simulink model "projectinitial-1"  (R2016a)
settings: Solver=VariableStepAuto  StartTime=0.0  StopTime=0.2  RelTol=1e-3
undefined symbols (not defined in the file): D1, Delta
libraries: powerlib x27, simulink_extras x2, dspsigops x2, powerlib_meascontrol x2
settings Model: Creator=Ejapistic Aamir  LastModifiedBy=Ejapistic Aamir

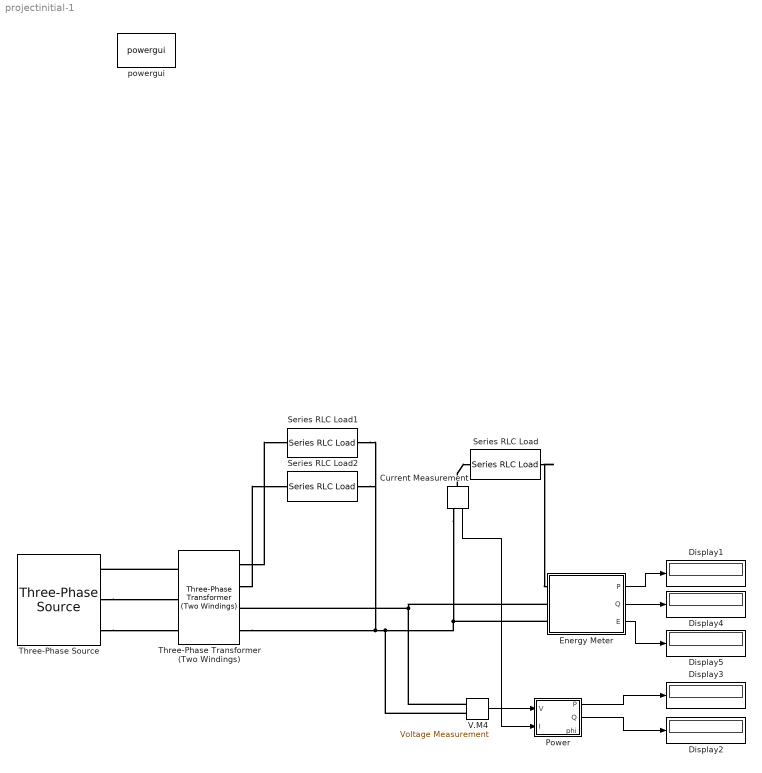
== system projectinitial-1 ==
  Current Measurement : powerlib/Measurements/Current Measurement  PhasorSimulation=off  OutputType=Complex  PSBequivalent=0
  Display{1..5} (5 alike) : Display
  Energy Meter : Subsystem
  Power : Subsystem  AncestorBlock=powerlib_meascontrol/Measurements/Power  DialogController=POWERSYS.PowerSysDialog  mask(Power){Freq=60, Vinit=[1, 0], Iinit=[1, 0], Ts=0}
      mask prompts: Freq "Fundamental frequency (Hz):"; Vinit "Voltage initial input [ Mag, Phase (degrees) ]:"; Iinit "Current initial input [ Mag, Phase (degrees) ]:"; Ts "Sample time:"
      mask help:
      | Compute the active and reactive powers of a voltage-current pair at fundamental frequency.
      |
      | For the first cycle of simulation, the outputs are held constant to the powers computed for the Voltage initial input and Current initial input parameters.
      mask init:
      | [WantBlockChoice,Ts,sps] = powericon('PowerInit',gcb,Freq,Vinit,Iinit,Ts);
      mask Help: helpview(psbhelp);
  Series RLC Load : powerlib/Elements/Series RLC Load  LConnTagsString=a  RConnTagsString=__new0  NominalVoltage=230  NominalFrequency=60  ActivePower=2000  InductivePower=700  CapacitivePower=00  Setx0=off  InitialVoltage=0  SetiL0=off  InitialCurrent=0  Measurements=None  LoadType=constant Z
  Series RLC Load1 : powerlib/Elements/Series RLC Load  LConnTagsString=a  RConnTagsString=__new0  NominalVoltage=100  NominalFrequency=60  ActivePower=1000  InductivePower=1000  CapacitivePower=00  Setx0=off  InitialVoltage=0  SetiL0=off  InitialCurrent=0  Measurements=None  LoadType=constant Z
  Series RLC Load2 : powerlib/Elements/Series RLC Load  LConnTagsString=a  RConnTagsString=__new0  NominalVoltage=100  NominalFrequency=60  ActivePower=1000  InductivePower=1000  CapacitivePower=00  Setx0=off  InitialVoltage=0  SetiL0=off  InitialCurrent=0  Measurements=None  LoadType=constant Z
  Three-Phase Transformer (Two Windings) : powerlib/Elements/Three-Phase Transformer (Two Windings)  Winding1Connection=Delta (D1)  Winding2Connection=Yn  CoreType=Three single-phase transformers  SetSaturation=off  Hysteresis=off  DataFile='hysteresis'  SetInitialFlux=off  Measurements=None  UNITS=pu  NominalPower=[ 250e6 , 60 ]  Winding1=[11000 , 0.002 , 0.08 ]  Winding2=[ 400 , 0.002 , 0.08 ]  Rm=501  Lm=500  L0=0.5  Saturation=[ 0,0 ; 0.0024,1.2 ; 1.0,1.52 ]  InitialFluxes=[ 0.8 , -0.8 , 0.7 ]  MoreParameters=off  BreakLoop=off  DataType=off  TransfoNumber=1
  Three-Phase Source : powerlib/Electrical Sources/Three-Phase Source  InternalConnection=Yg  VoltagePhases=off  Voltage=11000  PhaseAngle=0  Voltage_phases=[25e3 25e3 25e3]/sqrt(3)  PhaseAngles_phases=[0 -120 +120]  Frequency=60  NonIdealSource=on  SpecifyImpedance=off  Resistance=0.8929  Inductance=16.58e-3  ShortCircuitLevel=100e6  BaseVoltage=25e3  XRratio=7  BusType=swing  Pref=10e3  Qref=0  Prefabc=[10e3, 10e3, 10e3]  Qrefabc=[0, 0, 0]  Qmin=-inf  Qmax=inf
  V.M4 : powerlib/Measurements/Voltage Measurement  PhasorSimulation=off  OutputType=Complex  PSBequivalent=0
  powergui : powerlib/powergui  Priority=1  SimulationMode=Continuous  SolverType=Tustin/Backward Euler (TBE)  SampleTime=50e-6  frequency=60  SPID=off  DisableSnubberDevices=off  DisableRonSwitches=off  DisableVfSwitches=off  SwTol=0  DisplayEquations=off  Interpol=off  ExternalGateDelay=off  methode=off  Ts=10  FunctionMessages=off  echomessages=off  HookPort=off  EnableUseOfTLC=off  x0status=blocks  frequencyindice=60  Pbase=100e6  ErrMax=1e-4  Iterations=50  UnitsV=kV  UnitsW=MW  buscounter=0  RestoreLinks=warning  ResistiveCurrentMeasurement=off  Frange=[0:2:500]  Ylog=off  Xlog=on  ShowGrid=off  save=off  variable=ZData  structure=0  ZoomFFT=off  StartTime=0.0  cycles=1  DisplayStyle=1  fundamental=60  FreqAxis=off  MaxFrequency=1000  frequencyindicesteady=1  RmsSteady=1  display=off
  wires:
  V.M4/1 -> Power/1(V)
  Current Measurement/1 -> Power/2(I)
  Energy Meter/1(P) -> Display1/1
  Energy Meter/2(Q) -> Display4/1
  Power/1(P) -> Display3/1
  Power/2(Q) -> Display2/1
  Energy Meter/3(E) -> Display5/1
  connections:
  Three-Phase Transformer (Two Windings)/LConn1 -- Three-Phase Source/RConn1
  Three-Phase Source/RConn2 -- Three-Phase Transformer (Two Windings)/LConn2
  Three-Phase Source/RConn3 -- Three-Phase Transformer (Two Windings)/LConn3
  Three-Phase Transformer (Two Windings)/RConn1 -- Series RLC Load1/RConn1
  Three-Phase Transformer (Two Windings)/RConn2 -- Series RLC Load2/RConn1
  Current Measurement/LConn1 -- Series RLC Load/RConn1
  V.M4/LConn1 -- Energy Meter/LConn2 -- Three-Phase Transformer (Two Windings)/RConn3
  V.M4/LConn2 -- Three-Phase Transformer (Two Windings)/RConn4 -- Series RLC Load2/LConn1 -- Series RLC Load1/LConn1 -- Energy Meter/LConn3 -- Current Measurement/RConn1
  Series RLC Load/LConn1 -- Energy Meter/LConn1

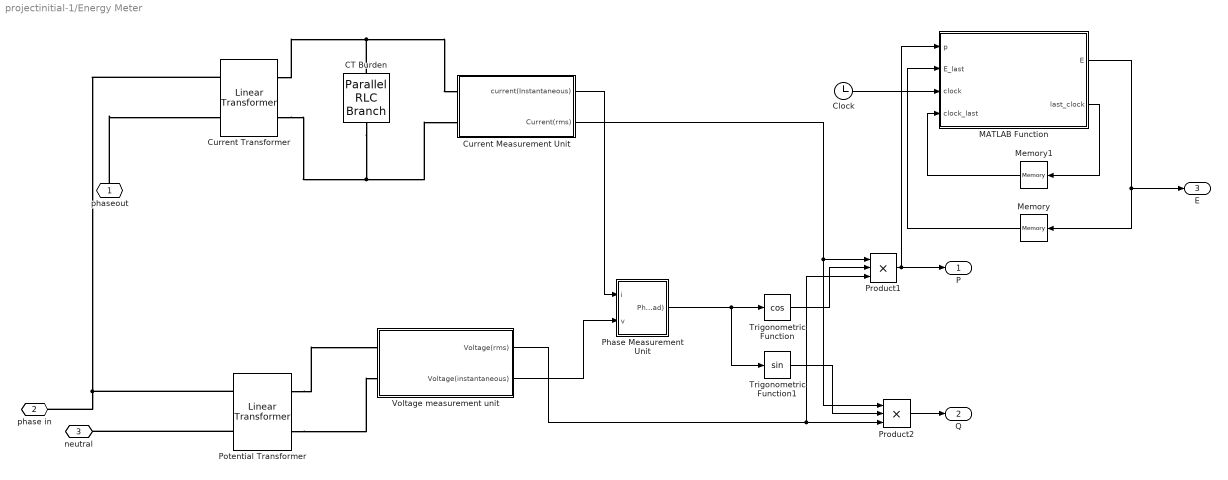
== system projectinitial-1/Energy Meter ==
  CT Burden : powerlib/Elements/Parallel RLC Branch  LConnTagsString=a  RConnTagsString=__new0  BranchType=R  Resistance=200  Inductance=0  SetiL0=off  InitialCurrent=0  Capacitance=1e-6  Setx0=off  InitialVoltage=0  Measurements=None
  Clock : Clock
  Current Measurement Unit : Subsystem
  Current Transformer : powerlib/Elements/Linear Transformer  UNITS=pu  NominalPower=[5 60 ]  winding1="[0.025  0.002  0.08 ]"  winding2="[15  0.002  0.08 ]"  ThreeWindings=off  winding3=[ 315e3 0.002 0.08 ]  RmLm=[ 500 500 ]  Measurements=None  DataType=off
  MATLAB Function : MATLAB Function  TreatAsAtomicUnit=on
  Memory : Memory
  Memory1 : Memory
  Phase Measurement Unit : Subsystem
  Potential Transformer : powerlib/Elements/Linear Transformer  UNITS=pu  NominalPower=[5 60 ]  winding1="[ 230  0.002  0.08 ]"  winding2="[ 5  0.002  0.08 ]"  ThreeWindings=off  winding3=[ 315e3 0.002 0.08 ]  RmLm=[ 500 500 ]  Measurements=None  DataType=off
  Product1 : Product  Inputs=3
  Product2 : Product  Inputs=3
  Trigonometric Function : Trigonometry  Operator=cos
  Trigonometric Function1 : Trigonometry
  Voltage measurement unit : Subsystem
  phaseout : PMIOPort  Port=1  Side=Left
  phase in : PMIOPort  Port=2  Side=Left
  neutral : PMIOPort  Port=3  Side=Left
  P : Outport
  Q : Outport  Port=2
  E : Outport  Port=3
  wires:
  Phase Measurement Unit/1(Phase (rad)) -> Trigonometric Function1/1, Trigonometric Function/1
  Current Measurement Unit/2(Current(rms)) -> Product2/1, Product1/1
  Voltage measurement unit/1(Voltage(rms)) -> Product2/3, Product1/3
  Current Measurement Unit/1(current(Instantaneous)) -> Phase Measurement Unit/1(i)
  Voltage measurement unit/2(Voltage(instantaneous)) -> Phase Measurement Unit/2(v)
  Product1/1 -> P/1, MATLAB Function/1(p)
  Trigonometric Function/1 -> Product1/2
  Trigonometric Function1/1 -> Product2/2
  Product2/1 -> Q/1
  MATLAB Function/1(E) -> Memory/1, E/1
  Memory/1 -> MATLAB Function/2(E_last)
  MATLAB Function/2(last_clock) -> Memory1/1
  Memory1/1 -> MATLAB Function/4(clock_last)
  Clock/1 -> MATLAB Function/3(clock)
  connections:
  Potential Transformer/LConn2 -- neutral/RConn1
  Potential Transformer/LConn1 -- phase in/RConn1 -- Current Transformer/LConn1
  phaseout/RConn1 -- Current Transformer/LConn2
  Current Transformer/RConn2 -- CT Burden/RConn1 -- Current Measurement Unit/LConn2
  Current Transformer/RConn1 -- CT Burden/LConn1 -- Current Measurement Unit/LConn1
  Potential Transformer/RConn2 -- Voltage measurement unit/LConn2
  Potential Transformer/RConn1 -- Voltage measurement unit/LConn1

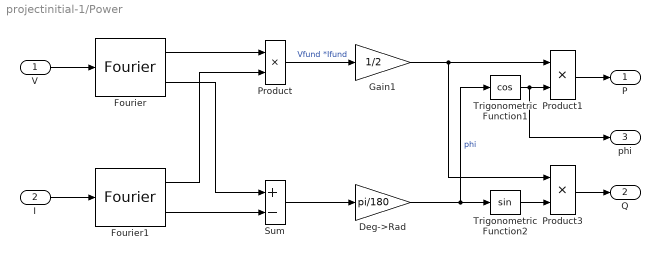
== system projectinitial-1/Power ==
  V : Inport  SampleTime=Ts
  I : Inport  Port=2  SampleTime=Ts
  Deg->Rad : Gain  Gain=pi/180  SaturateOnIntegerOverflow=on  OutDataTypeStr=Inherit: Same as input  ParamDataTypeStr=Inherit: Same as input
  Fourier : powerlib_meascontrol/Measurements/Fourier  Freq=sps.Freq  n=1  InInit=sps.Par_Vinit  Ts=Ts
  Fourier1 : powerlib_meascontrol/Measurements/Fourier  Freq=sps.Freq  n=1  InInit=sps.Par_Iinit  Ts=Ts
  Gain1 : Gain  Gain=1/2  SaturateOnIntegerOverflow=on  OutDataTypeStr=Inherit: Same as input  ParamDataTypeStr=Inherit: Same as input
  Product : Product  SaturateOnIntegerOverflow=on  InputSameDT=on  OutDataTypeStr=Inherit: Same as first input
  Product1 : Product  SaturateOnIntegerOverflow=on  InputSameDT=on  OutDataTypeStr=Inherit: Same as first input
  Product3 : Product  SaturateOnIntegerOverflow=on  InputSameDT=on  OutDataTypeStr=Inherit: Same as first input
  Sum : Sum  Inputs=+-  SaturateOnIntegerOverflow=on  InputSameDT=on  OutDataTypeStr=Inherit: Same as first input
  Trigonometric Function1 : Trigonometry  Operator=cos
  Trigonometric Function2 : Trigonometry
  P : Outport  SampleTime=Ts
  Q : Outport  Port=2  SampleTime=Ts
  phi : Outport  Port=3  SampleTime=Ts
  wires:
  Gain1/1 -> Product3/1, Product1/1
  Product3/1 -> Q/1
  Fourier1/2 -> Sum/2
  Fourier/2 -> Sum/1
  Deg->Rad/1 -> Trigonometric Function2/1, Trigonometric Function1/1  "phi"
  Trigonometric Function2/1 -> Product3/2
  Product/1 -> Gain1/1  "Vfund *Ifund"
  V/1 -> Fourier/1
  I/1 -> Fourier1/1
  Sum/1 -> Deg->Rad/1
  Trigonometric Function1/1 -> phi/1, Product1/2
  Fourier/1 -> Product/1
  Fourier1/1 -> Product/2
  Product1/1 -> P/1

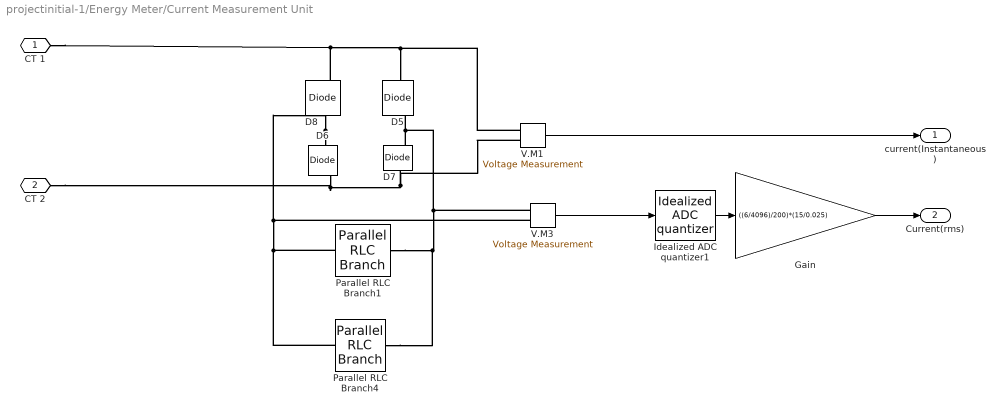
== system projectinitial-1/Energy Meter/Current Measurement Unit ==
  D{5..8} (4 alike) : powerlib/Power Electronics/Diode  Ron=0.001  Lon=0  Vf=0.3  IC=0  UseSnubber=off  Rs=500  Cs=250e-9  Measurements=on
  Gain : Gain  Gain=((6/4096)/200)*(15/0.025)
  Idealized ADC quantizer1 : simulink_extras/Additional Discrete/Idealized ADC quantizer  NumberOfConverterBits=12  Vmin=0  Vmax=6  OutputDataType=uint32  OutputNegativeValues=off
  Parallel RLC Branch1 : powerlib/Elements/Parallel RLC Branch  LConnTagsString=a  RConnTagsString=__new0  BranchType=R  Resistance=26000  Inductance=0  SetiL0=off  InitialCurrent=0  Capacitance=1e-6  Setx0=off  InitialVoltage=0  Measurements=None
  Parallel RLC Branch4 : powerlib/Elements/Parallel RLC Branch  LConnTagsString=a  RConnTagsString=__new0  BranchType=C  Resistance=0  Inductance=0  SetiL0=off  InitialCurrent=0  Capacitance=1e-5  Setx0=off  InitialVoltage=0  Measurements=None
  V.M1 : powerlib/Measurements/Voltage Measurement  PhasorSimulation=off  OutputType=Complex  PSBequivalent=0
  V.M3 : powerlib/Measurements/Voltage Measurement  PhasorSimulation=off  OutputType=Complex  PSBequivalent=0
  CT 1 : PMIOPort  Port=1  Side=Left
  CT 2 : PMIOPort  Port=2  Side=Left
  current(Instantaneous) : Outport
  Current(rms) : Outport  Port=2
  wires:
  V.M1/1 -> current(Instantaneous)/1
  Idealized ADC quantizer1/1 -> Gain/1
  Gain/1 -> Current(rms)/1
  V.M3/1 -> Idealized ADC quantizer1/1
  connections:
  D7/RConn1 -- Parallel RLC Branch4/LConn1 -- Parallel RLC Branch1/RConn1 -- V.M3/LConn1 -- D5/RConn1
  D6/RConn1 -- CT 2/RConn1 -- V.M1/LConn2 -- D7/LConn1
  D8/LConn1 -- Parallel RLC Branch4/RConn1 -- Parallel RLC Branch1/LConn1 -- V.M3/LConn2 -- D6/LConn1
  D8/RConn1 -- CT 1/RConn1 -- V.M1/LConn1 -- D5/LConn1

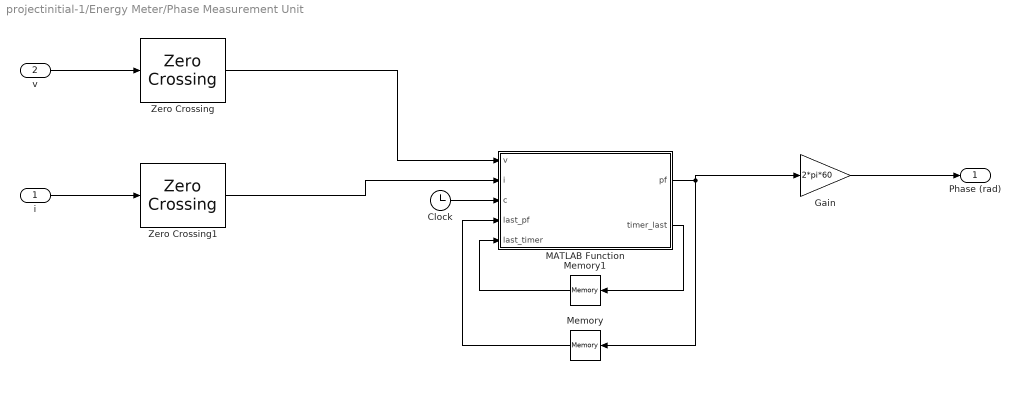
== system projectinitial-1/Energy Meter/Phase Measurement Unit ==
  i : Inport
  v : Inport  Port=2
  Clock : Clock
      settings: Decimation=1000
  Gain : Gain  Gain=2*pi*60  OutDataTypeStr=double
  MATLAB Function : MATLAB Function  TreatAsAtomicUnit=on
  Memory : Memory
  Memory1 : Memory
  Zero Crossing : dspsigops/Zero Crossing  InputProcessing=Columns as channels (frame based)
  Zero Crossing1 : dspsigops/Zero Crossing  InputProcessing=Columns as channels (frame based)
  Phase (rad) : Outport
  wires:
  Clock/1 -> MATLAB Function/3(c)
  v/1 -> Zero Crossing/1
  i/1 -> Zero Crossing1/1
  Zero Crossing1/1 -> MATLAB Function/2(i)
  Zero Crossing/1 -> MATLAB Function/1(v)
  MATLAB Function/1(pf) -> Gain/1, Memory/1
  Memory1/1 -> MATLAB Function/5(last_timer)
  MATLAB Function/2(timer_last) -> Memory1/1
  Memory/1 -> MATLAB Function/4(last_pf)
  Gain/1 -> Phase (rad)/1

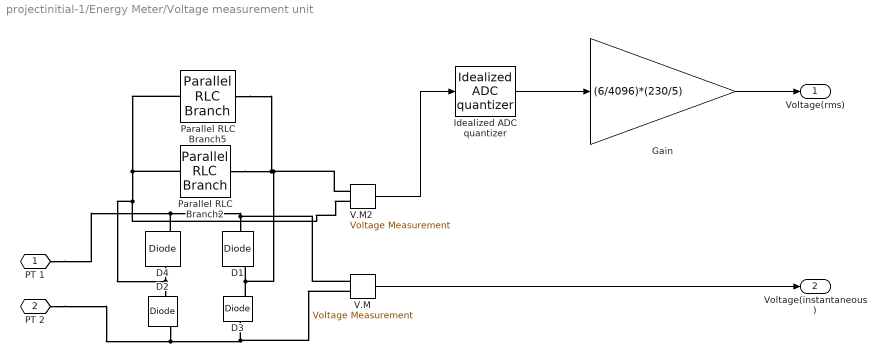
== system projectinitial-1/Energy Meter/Voltage measurement unit ==
  D{1..4} (4 alike) : powerlib/Power Electronics/Diode  Ron=0.001  Lon=0  Vf=1  IC=0  UseSnubber=off  Rs=500  Cs=250e-9  Measurements=on
  Gain : Gain  Gain=(6/4096)*(230/5)
  Idealized ADC quantizer : simulink_extras/Additional Discrete/Idealized ADC quantizer  NumberOfConverterBits=12  Vmin=0  Vmax=6  OutputDataType=uint32  OutputNegativeValues=off
  Parallel RLC Branch2 : powerlib/Elements/Parallel RLC Branch  LConnTagsString=a  RConnTagsString=__new0  BranchType=C  Resistance=0  Inductance=0  SetiL0=off  InitialCurrent=0  Capacitance=1e-5  Setx0=off  InitialVoltage=0  Measurements=None
  Parallel RLC Branch5 : powerlib/Elements/Parallel RLC Branch  LConnTagsString=a  RConnTagsString=__new0  BranchType=R  Resistance=26000  Inductance=0  SetiL0=off  InitialCurrent=0  Capacitance=1e-6  Setx0=off  InitialVoltage=0  Measurements=None
  V.M : powerlib/Measurements/Voltage Measurement  PhasorSimulation=off  OutputType=Complex  PSBequivalent=0
  V.M2 : powerlib/Measurements/Voltage Measurement  PhasorSimulation=off  OutputType=Complex  PSBequivalent=0
  PT 1 : PMIOPort  Port=1  Side=Left
  PT 2 : PMIOPort  Port=2  Side=Left
  Voltage(rms) : Outport
  Voltage(instantaneous) : Outport  Port=2
  wires:
  V.M2/1 -> Idealized ADC quantizer/1
  V.M/1 -> Voltage(instantaneous)/1
  Idealized ADC quantizer/1 -> Gain/1
  Gain/1 -> Voltage(rms)/1
  connections:
  D4/RConn1 -- PT 1/RConn1 -- V.M/LConn1 -- D1/LConn1
  D3/RConn1 -- V.M2/LConn1 -- Parallel RLC Branch2/LConn1 -- Parallel RLC Branch5/RConn1 -- D1/RConn1
  D4/LConn1 -- Parallel RLC Branch5/LConn1 -- Parallel RLC Branch2/RConn1 -- V.M2/LConn2 -- D2/LConn1
  D2/RConn1 -- PT 2/RConn1 -- V.M/LConn2 -- D3/LConn1

== matlab function projectinitial-1/Energy Meter/MATLAB Function ==
  data: p input; E output; E_last input; clock input; clock_last input; last_clock output
function [E,last_clock] = Energy_Measurement(p,E_last,clock,clock_last)
%#codegen
a=clock;
E=E_last+p*(a-clock_last)/(1000*60*60);
last_clock=[a];
E = [E];

== matlab function projectinitial-1/Energy Meter/Phase Measurement Unit/MATLAB Function ==
  data: v input; pf output; i input; c input; last_pf input; last_timer input; timer_last output
function [pf,timer_last] =pf_measurement(v,i,c,last_pf,last_timer)

if v==1
    timer_now=c;
    
else
    timer_now=last_timer;
end
if i==1
    timer_old=timer_now;
    timer_now=c;
    pf=timer_now-timer_old;
    pf=[pf];
    last_pf=pf;
else
    pf=[last_pf];
end
timer_last=[timer_now];

end
